simulink model "foc"  (Simulink 5.0)
settings: Solver=ode5  StartTime=0.0  StopTime=3  FixedStep=0.00001  RelTol=1e-3
settings Model: LastModifiedBy=Administrator

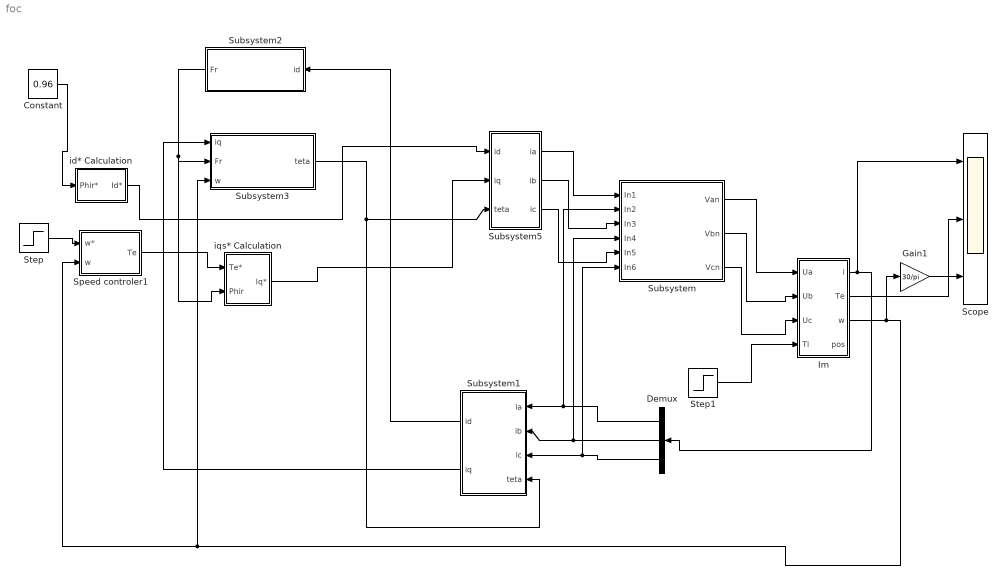
== system foc ==
  Constant : Constant  Value=0.96
  Demux : Demux  Orientation=left  Outputs=3
  Gain1 : Gain  Gain=30/pi  SaturateOnIntegerOverflow=on
  Im : Subsystem  mask{Rs=4.1, Rr=2.5, Ls=0.545, Lr=0.542, Lm=0.510, J=0.04, p=2, Lsc=0.065}
      mask prompts: Rs "stator r(Rs)"; Rr "rotor r(Rr)"; Ls "stator l(Ls)"; Lr "rotor l(Lr)"; Lm "s r l(Lm)"; J "z(J)"; p "jiduishu(p)"; Lsc "l(Lsc)"
  Scope : Scope  NumInputPorts=3
      settings: TimeRange=3  YMin=-12.5~-15~500  YMax=12.5~15~2500  MaxDataPoints=5000000
  Speed controler1 : Subsystem  mask{Kp=30, Ki=5}
  Step : Step  Before=250  After=150  SampleTime=0
  Step1 : Step  Time=2  After=5  SampleTime=0
  Subsystem : Subsystem  mask{Vd=780}
  Subsystem1 : Subsystem  Orientation=left
  Subsystem2 : Subsystem  Orientation=left  mask{Lr=0.542, Lm=0.510, Rr=2.5}
  Subsystem3 : Subsystem  mask{Lr=0.542, Lm=0.510, Rr=2.5}
  Subsystem5 : Subsystem
  id* Calculation : Subsystem
  iqs* Calculation : Subsystem
  wires:
  Demux/1 -> Subsystem1/1(ia), Subsystem/2(In2)
  Demux/2 -> Subsystem1/2(ib), Subsystem/4(In4)
  Demux/3 -> Subsystem1/3(ic), Subsystem/6(In6)
  Subsystem2/1(Fr) -> Subsystem3/2(Fr), iqs* Calculation/2(Phir)
  Subsystem1/2(iq) -> Subsystem3/1(iq)
  Subsystem1/1(id) -> Subsystem2/1(id)
  Subsystem3/1(teta) -> Subsystem1/4(teta), Subsystem5/3(teta)
  iqs* Calculation/1(Iq*) -> Subsystem5/2(iq)
  Subsystem5/1(ia) -> Subsystem/1(In1)
  Subsystem5/2(ib) -> Subsystem/3(In3)
  Subsystem5/3(ic) -> Subsystem/5(In5)
  Subsystem/1(Van) -> Im/1(Ua)
  Subsystem/2(Vbn) -> Im/2(Ub)
  Subsystem/3(Vcn) -> Im/3(Uc)
  Im/3(w) -> Subsystem3/3(w), Speed controler1/2(w), Gain1/1
  Im/1(i) -> Demux/1, Scope/1
  Constant/1 -> id* Calculation/1(Phir*)
  id* Calculation/1(Id*) -> Subsystem5/1(id)
  Step/1 -> Speed controler1/1(w*)
  Im/2(Te) -> Scope/2
  Step1/1 -> Im/4(Tl)
  Speed controler1/1(Te) -> iqs* Calculation/1(Te*)
  Gain1/1 -> Scope/3

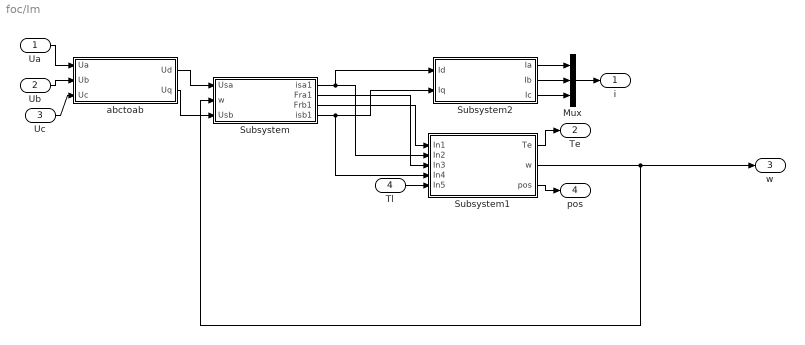
== system foc/Im ==
  Ua : Inport
  Ub : Inport  Port=2
  Uc : Inport  Port=3
  Tl : Inport  Port=4
  Mux : Mux  Inputs=3
  Subsystem : Subsystem
  Subsystem1 : Subsystem
  Subsystem2 : Subsystem
  abctoab : Subsystem
  i : Outport
  Te : Outport  Port=2
  w : Outport  Port=3
  pos : Outport  Port=4
  wires:
  Ua/1 -> abctoab/1(Ua)
  Mux/1 -> i/1
  Ub/1 -> abctoab/2(Ub)
  Uc/1 -> abctoab/3(Uc)
  Subsystem1/1(Te) -> Te/1
  Tl/1 -> Subsystem1/5(In5)
  Subsystem1/3(pos) -> pos/1
  Subsystem1/2(w) -> Subsystem/2(w), w/1
  Subsystem2/3(Ic) -> Mux/3
  Subsystem2/2(Ib) -> Mux/2
  Subsystem2/1(Ia) -> Mux/1
  Subsystem/2(Fra1) -> Subsystem1/3(In3)
  Subsystem/3(Frb1) -> Subsystem1/1(In1)
  Subsystem/4(isb1) -> Subsystem2/2(Iq), Subsystem1/4(In4)
  Subsystem/1(isa1) -> Subsystem2/1(Id), Subsystem1/2(In2)
  abctoab/2(Uq) -> Subsystem/3(Usb)
  abctoab/1(Ud) -> Subsystem/1(Usa)

== system foc/Speed controler1 ==
  w* : Inport
  w : Inport  Port=2
  Gain : Gain  Gain=Kp  SaturateOnIntegerOverflow=on
  Gain1 : Gain  Gain=Ki  SaturateOnIntegerOverflow=on
  Integrator : Integrator
  Saturation : Saturate  UpperLimit=20  LowerLimit=-20
  Sum : Sum  Inputs=|+-  SaturateOnIntegerOverflow=on
  Sum1 : Sum  Inputs=|++  SaturateOnIntegerOverflow=on
  Te : Outport
  wires:
  Sum/1 -> Gain/1, Gain1/1
  Gain1/1 -> Integrator/1
  Integrator/1 -> Sum1/2
  Gain/1 -> Sum1/1
  w*/1 -> Sum/1
  w/1 -> Sum/2
  Sum1/1 -> Saturation/1
  Saturation/1 -> Te/1

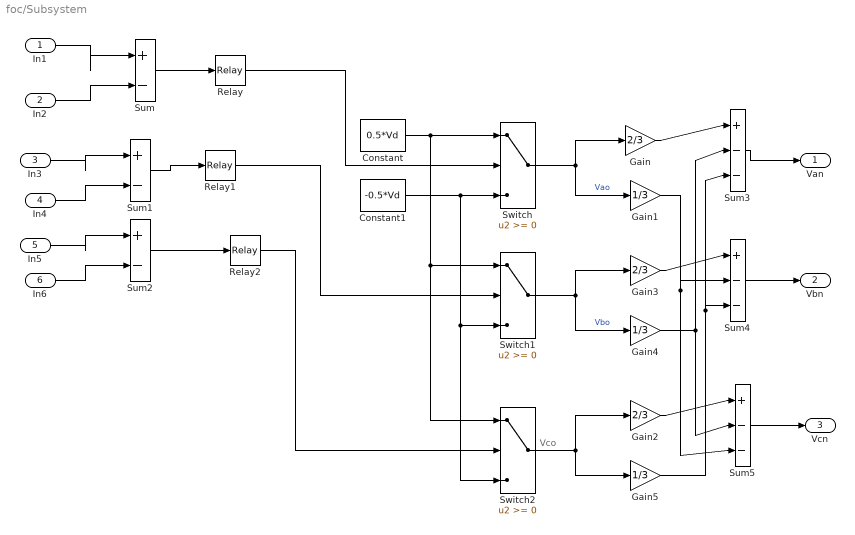
== system foc/Subsystem ==
  note: Vco
  In1 : Inport
  In2 : Inport  Port=2
  In3 : Inport  Port=3
  In4 : Inport  Port=4
  In5 : Inport  Port=5
  In6 : Inport  Port=6
  Constant : Constant  Value=0.5*Vd
  Constant1 : Constant  Value=-0.5*Vd
  Gain : Gain  Gain=2/3  SaturateOnIntegerOverflow=on
  Gain1 : Gain  Gain=1/3  SaturateOnIntegerOverflow=on
  Gain2 : Gain  Gain=2/3  SaturateOnIntegerOverflow=on
  Gain3 : Gain  Gain=2/3  SaturateOnIntegerOverflow=on
  Gain4 : Gain  Gain=1/3  SaturateOnIntegerOverflow=on
  Gain5 : Gain  Gain=1/3  SaturateOnIntegerOverflow=on
  Relay : Relay  OnSwitchValue=0.001  OffSwitchValue=-0.001  OffOutputValue=-1
  Relay1 : Relay  OnSwitchValue=0.001  OffSwitchValue=0.001  OffOutputValue=-1
  Relay2 : Relay  OnSwitchValue=0.001  OffSwitchValue=0.001  OffOutputValue=-1
  Sum : Sum  Inputs=|+-  SaturateOnIntegerOverflow=on
  Sum1 : Sum  Inputs=|+-  SaturateOnIntegerOverflow=on
  Sum2 : Sum  Inputs=|+-  SaturateOnIntegerOverflow=on
  Sum3 : Sum  Inputs=|+--  SaturateOnIntegerOverflow=on
  Sum4 : Sum  Inputs=|+--  SaturateOnIntegerOverflow=on
  Sum5 : Sum  Inputs=|+--  SaturateOnIntegerOverflow=on
  Switch : Switch  SaturateOnIntegerOverflow=on
  Switch1 : Switch  SaturateOnIntegerOverflow=on
  Switch2 : Switch  SaturateOnIntegerOverflow=on
  Van : Outport
  Vbn : Outport  Port=2
  Vcn : Outport  Port=3
  wires:
  Sum/1 -> Relay/1
  In1/1 -> Sum/1
  In2/1 -> Sum/2
  In3/1 -> Sum1/1
  In4/1 -> Sum1/2
  In5/1 -> Sum2/1
  In6/1 -> Sum2/2
  Sum2/1 -> Relay2/1
  Sum1/1 -> Relay1/1
  Relay/1 -> Switch/2
  Constant/1 -> Switch/1, Switch2/1, Switch1/1
  Constant1/1 -> Switch/3, Switch2/3, Switch1/3
  Switch/1 -> Gain/1, Gain1/1  "Vao"
  Switch1/1 -> Gain3/1, Gain4/1  "Vbo"
  Switch2/1 -> Gain2/1, Gain5/1
  Sum3/1 -> Van/1
  Sum4/1 -> Vbn/1
  Sum5/1 -> Vcn/1
  Gain/1 -> Sum3/1
  Gain4/1 -> Sum3/2, Sum5/2
  Gain5/1 -> Sum3/3, Sum4/3
  Gain3/1 -> Sum4/1
  Gain1/1 -> Sum4/2, Sum5/3
  Gain2/1 -> Sum5/1
  Relay1/1 -> Switch1/2
  Relay2/1 -> Switch2/2

== system foc/Subsystem1 ==
  ia : Inport
  ib : Inport  Port=2
  ic : Inport  Port=3
  teta : Inport  Port=4
  VR : Subsystem
  abctoab : Subsystem
  id : Outport
  iq : Outport  Port=2
  wires:
  VR/2(Out2) -> iq/1
  VR/1(Out1) -> id/1
  teta/1 -> VR/3(In3)
  ic/1 -> abctoab/3(Uc)
  ib/1 -> abctoab/2(Ub)
  ia/1 -> abctoab/1(Ua)
  abctoab/2(Uq) -> VR/2(In2)
  abctoab/1(Ud) -> VR/1(In1)

== system foc/Subsystem2 ==
  id : Inport
  Gain : Gain  Gain=Lm*Rr  SaturateOnIntegerOverflow=on
  Transfer Fcn : TransferFcn  Denominator=[Lr Rr]
  Fr : Outport
  wires:
  Transfer Fcn/1 -> Fr/1
  Gain/1 -> Transfer Fcn/1
  id/1 -> Gain/1

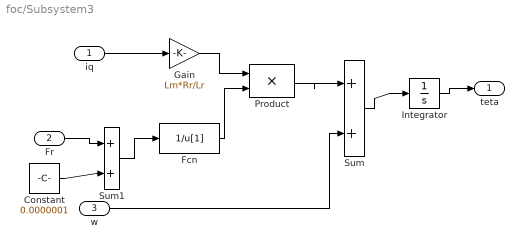
== system foc/Subsystem3 ==
  iq : Inport
  Fr : Inport  Port=2
  w : Inport  Port=3
  Constant : Constant  Value=0.0000001
  Fcn : Fcn  Expr=1/u[1]
  Gain : Gain  Gain=Lm*Rr/Lr  SaturateOnIntegerOverflow=on
  Integrator : Integrator
  Product : Product  SaturateOnIntegerOverflow=on
  Sum : Sum  Inputs=|++  SaturateOnIntegerOverflow=on
  Sum1 : Sum  Inputs=|++  SaturateOnIntegerOverflow=on
  teta : Outport
  wires:
  Product/1 -> Sum/1
  Fcn/1 -> Product/2
  Gain/1 -> Product/1
  iq/1 -> Gain/1
  Sum/1 -> Integrator/1
  Integrator/1 -> teta/1
  w/1 -> Sum/2
  Constant/1 -> Sum1/2
  Fr/1 -> Sum1/1
  Sum1/1 -> Fcn/1

== system foc/Subsystem5 ==
  id : Inport
  iq : Inport  Port=2
  teta : Inport  Port=3
  Subsystem2 : Subsystem
  VR-1 : Subsystem
  ia : Outport
  ib : Outport  Port=2
  ic : Outport  Port=3
  wires:
  Subsystem2/3(Ic) -> ic/1
  Subsystem2/2(Ib) -> ib/1
  Subsystem2/1(Ia) -> ia/1
  teta/1 -> VR-1/3(teta)
  iq/1 -> VR-1/2(iq)
  id/1 -> VR-1/1(id)
  VR-1/2(ib) -> Subsystem2/2(Iq)
  VR-1/1(ia) -> Subsystem2/1(Id)

== system foc/id* Calculation ==
  note: Id* = Phir*/ Lm
  note: Lm= 34.7 mH
  Phir* : Inport
  KF : Gain  Gain=1/0.51  SaturateOnIntegerOverflow=on
  Id* : Outport
  wires:
  KF/1 -> Id*/1
  Phir*/1 -> KF/1

== system foc/iqs* Calculation ==
  note: Iq= ( 2/3) * (2/p) * ( Lr/Lm) * (Te / Phir)
  note: Lm = 34.7 mH
  note: Lr = Ll'r +Lm = 0.8 +34.7= 35.5 mH
  note: p= nb of poles = 4
  note: Iq= 0.341 * (Te / Phir)
  Te* : Inport
  Phir : Inport  Port=2
  Fcn : Fcn  Expr=u[1]*0.341/(u[2]+1e-3)
  Mux1 : Mux  Inputs=2
  Iq* : Outport  InitialOutput=0
  wires:
  Phir/1 -> Mux1/2
  Fcn/1 -> Iq*/1
  Te*/1 -> Mux1/1
  Mux1/1 -> Fcn/1

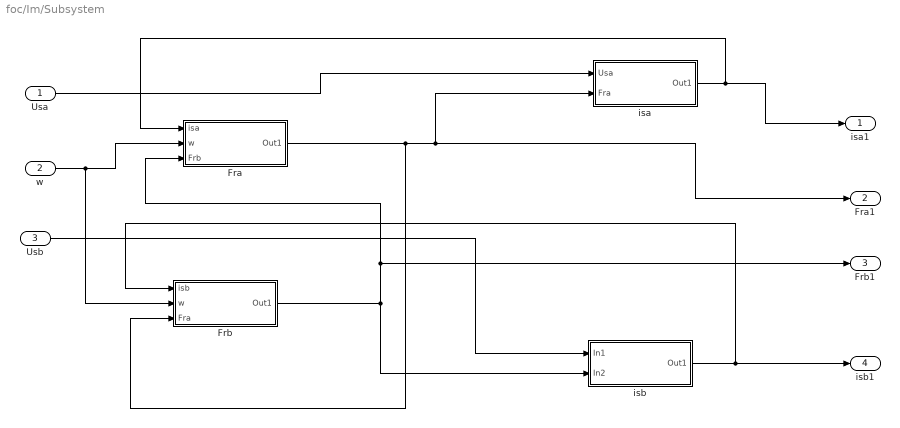
== system foc/Im/Subsystem ==
  Usa : Inport
  w : Inport  Port=2
  Usb : Inport  Port=3
  Fra : Subsystem
  Frb : Subsystem
  isa : Subsystem
  isb : Subsystem
  isa1 : Outport
  Fra1 : Outport  Port=2
  Frb1 : Outport  Port=3
  isb1 : Outport  Port=4
  wires:
  Usa/1 -> isa/1(Usa)
  Fra/1(Out1) -> Frb/3(Fra), isa/2(Fra), Fra1/1
  isa/1(Out1) -> isa1/1, Fra/1(isa)
  w/1 -> Fra/2(w), Frb/2(w)
  Frb/1(Out1) -> isb/2(In2), Fra/3(Frb), Frb1/1
  Usb/1 -> isb/1(In1)
  isb/1(Out1) -> Frb/1(isb), isb1/1

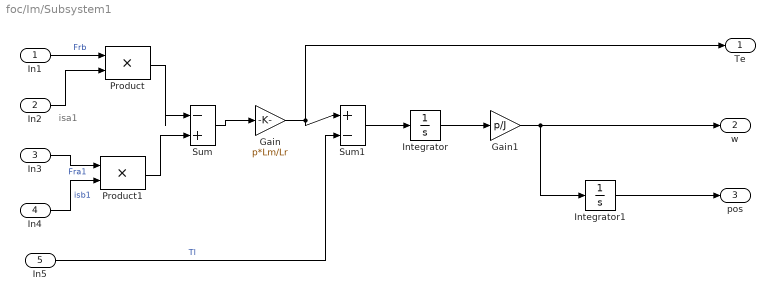
== system foc/Im/Subsystem1 ==
  note: isa1
  In1 : Inport
  In2 : Inport  Port=2
  In3 : Inport  Port=3
  In4 : Inport  Port=4
  In5 : Inport  Port=5
  Gain : Gain  Gain=p*Lm/Lr  SaturateOnIntegerOverflow=on
  Gain1 : Gain  Gain=p/J  SaturateOnIntegerOverflow=on
  Integrator : Integrator
  Integrator1 : Integrator
  Product : Product  SaturateOnIntegerOverflow=on
  Product1 : Product  SaturateOnIntegerOverflow=on
  Sum : Sum  Inputs=|-+  SaturateOnIntegerOverflow=on
  Sum1 : Sum  Inputs=|+-  SaturateOnIntegerOverflow=on
  Te : Outport
  w : Outport  Port=2
  pos : Outport  Port=3
  wires:
  In1/1 -> Product/1  "Frb"
  In2/1 -> Product/2
  In3/1 -> Product1/1  "Fra1"
  In4/1 -> Product1/2  "isb1"
  Product/1 -> Sum/1
  Product1/1 -> Sum/2
  Sum/1 -> Gain/1
  Gain/1 -> Sum1/1, Te/1
  In5/1 -> Sum1/2  "Tl"
  Sum1/1 -> Integrator/1
  Integrator/1 -> Gain1/1
  Gain1/1 -> w/1, Integrator1/1
  Integrator1/1 -> pos/1

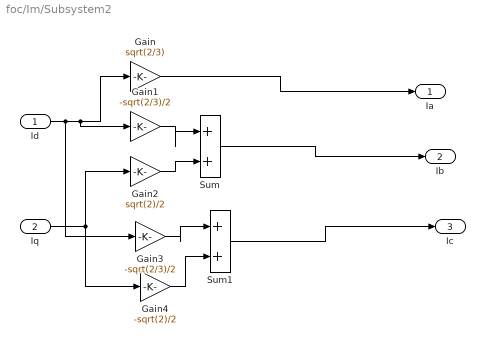
== system foc/Im/Subsystem2 ==
  Id : Inport
  Iq : Inport  Port=2
  Gain : Gain  Gain=sqrt(2/3)  SaturateOnIntegerOverflow=on
  Gain1 : Gain  Gain=-sqrt(2/3)/2  SaturateOnIntegerOverflow=on
  Gain2 : Gain  Gain=sqrt(2)/2  SaturateOnIntegerOverflow=on
  Gain3 : Gain  Gain=-sqrt(2/3)/2  SaturateOnIntegerOverflow=on
  Gain4 : Gain  Gain=-sqrt(2)/2  SaturateOnIntegerOverflow=on
  Sum : Sum  Inputs=|++  SaturateOnIntegerOverflow=on
  Sum1 : Sum  Inputs=|++  SaturateOnIntegerOverflow=on
  Ia : Outport
  Ib : Outport  Port=2
  Ic : Outport  Port=3
  wires:
  Sum1/1 -> Ic/1
  Gain4/1 -> Sum1/2
  Gain3/1 -> Sum1/1
  Sum/1 -> Ib/1
  Gain2/1 -> Sum/2
  Gain1/1 -> Sum/1
  Iq/1 -> Gain4/1, Gain2/1
  Gain/1 -> Ia/1
  Id/1 -> Gain3/1, Gain1/1, Gain/1

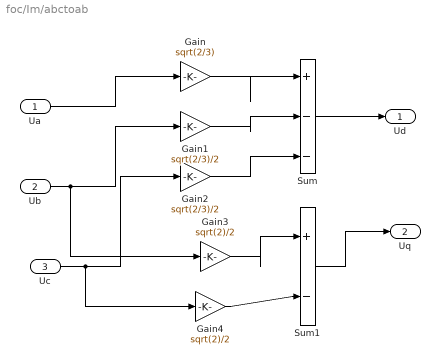
== system foc/Im/abctoab ==
  Ua : Inport
  Ub : Inport  Port=2
  Uc : Inport  Port=3
  Gain : Gain  Gain=sqrt(2/3)  SaturateOnIntegerOverflow=on
  Gain1 : Gain  Gain=sqrt(2/3)/2  SaturateOnIntegerOverflow=on
  Gain2 : Gain  Gain=sqrt(2/3)/2  SaturateOnIntegerOverflow=on
  Gain3 : Gain  Gain=sqrt(2)/2  SaturateOnIntegerOverflow=on
  Gain4 : Gain  Gain=sqrt(2)/2  SaturateOnIntegerOverflow=on
  Sum : Sum  Inputs=|+--  SaturateOnIntegerOverflow=on
  Sum1 : Sum  Inputs=|+-  SaturateOnIntegerOverflow=on
  Ud : Outport
  Uq : Outport  Port=2
  wires:
  Sum1/1 -> Uq/1
  Gain4/1 -> Sum1/2
  Gain3/1 -> Sum1/1
  Sum/1 -> Ud/1
  Gain2/1 -> Sum/3
  Gain1/1 -> Sum/2
  Gain/1 -> Sum/1
  Uc/1 -> Gain4/1, Gain2/1
  Ub/1 -> Gain3/1, Gain1/1
  Ua/1 -> Gain/1

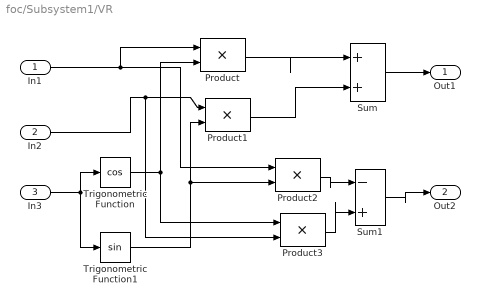
== system foc/Subsystem1/VR ==
  In1 : Inport
  In2 : Inport  Port=2
  In3 : Inport  Port=3
  Product{,1..3} (4 alike) : Product  SaturateOnIntegerOverflow=on
  Sum : Sum  Inputs=|++  SaturateOnIntegerOverflow=on
  Sum1 : Sum  Inputs=|-+  SaturateOnIntegerOverflow=on
  Trigonometric Function : Trigonometry  Operator=cos
  Trigonometric Function1 : Trigonometry
  Out1 : Outport
  Out2 : Outport  Port=2
  wires:
  Product3/1 -> Sum1/2
  Product2/1 -> Sum1/1
  Product1/1 -> Sum/2
  In2/1 -> Product3/2, Product1/1
  Trigonometric Function1/1 -> Product2/2, Product1/2
  Product/1 -> Sum/1
  Trigonometric Function/1 -> Product3/1, Product/2
  In1/1 -> Product2/1, Product/1
  Sum1/1 -> Out2/1
  In3/1 -> Trigonometric Function1/1, Trigonometric Function/1
  Sum/1 -> Out1/1

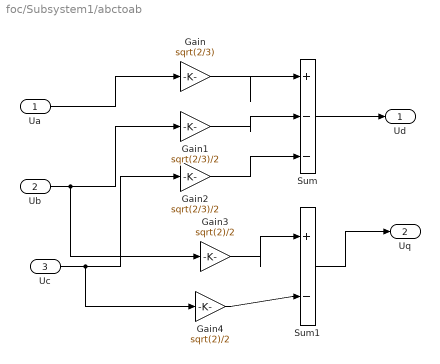
== system foc/Subsystem1/abctoab ==
  Ua : Inport
  Ub : Inport  Port=2
  Uc : Inport  Port=3
  Gain : Gain  Gain=sqrt(2/3)  SaturateOnIntegerOverflow=on
  Gain1 : Gain  Gain=sqrt(2/3)/2  SaturateOnIntegerOverflow=on
  Gain2 : Gain  Gain=sqrt(2/3)/2  SaturateOnIntegerOverflow=on
  Gain3 : Gain  Gain=sqrt(2)/2  SaturateOnIntegerOverflow=on
  Gain4 : Gain  Gain=sqrt(2)/2  SaturateOnIntegerOverflow=on
  Sum : Sum  Inputs=|+--  SaturateOnIntegerOverflow=on
  Sum1 : Sum  Inputs=|+-  SaturateOnIntegerOverflow=on
  Ud : Outport
  Uq : Outport  Port=2
  wires:
  Sum1/1 -> Uq/1
  Gain4/1 -> Sum1/2
  Gain3/1 -> Sum1/1
  Sum/1 -> Ud/1
  Gain2/1 -> Sum/3
  Gain1/1 -> Sum/2
  Gain/1 -> Sum/1
  Uc/1 -> Gain4/1, Gain2/1
  Ub/1 -> Gain3/1, Gain1/1
  Ua/1 -> Gain/1

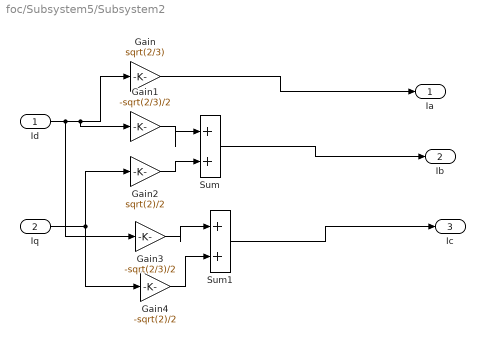
== system foc/Subsystem5/Subsystem2 ==
  Id : Inport
  Iq : Inport  Port=2
  Gain : Gain  Gain=sqrt(2/3)  SaturateOnIntegerOverflow=on
  Gain1 : Gain  Gain=-sqrt(2/3)/2  SaturateOnIntegerOverflow=on
  Gain2 : Gain  Gain=sqrt(2)/2  SaturateOnIntegerOverflow=on
  Gain3 : Gain  Gain=-sqrt(2/3)/2  SaturateOnIntegerOverflow=on
  Gain4 : Gain  Gain=-sqrt(2)/2  SaturateOnIntegerOverflow=on
  Sum : Sum  Inputs=|++  SaturateOnIntegerOverflow=on
  Sum1 : Sum  Inputs=|++  SaturateOnIntegerOverflow=on
  Ia : Outport
  Ib : Outport  Port=2
  Ic : Outport  Port=3
  wires:
  Id/1 -> Gain/1, Gain1/1, Gain3/1
  Gain/1 -> Ia/1
  Iq/1 -> Gain2/1, Gain4/1
  Gain1/1 -> Sum/1
  Gain2/1 -> Sum/2
  Sum/1 -> Ib/1
  Gain3/1 -> Sum1/1
  Gain4/1 -> Sum1/2
  Sum1/1 -> Ic/1

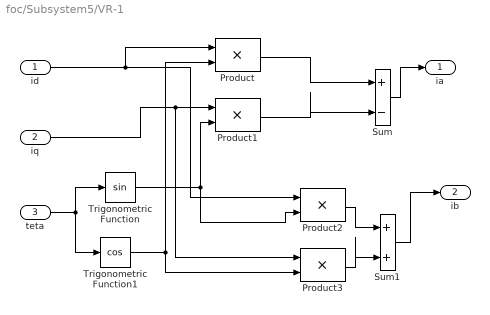
== system foc/Subsystem5/VR-1 ==
  id : Inport
  iq : Inport  Port=2
  teta : Inport  Port=3
  Product{,1..3} (4 alike) : Product  SaturateOnIntegerOverflow=on
  Sum : Sum  Inputs=|+-  SaturateOnIntegerOverflow=on
  Sum1 : Sum  Inputs=|++  SaturateOnIntegerOverflow=on
  Trigonometric Function : Trigonometry
  Trigonometric Function1 : Trigonometry  Operator=cos
  ia : Outport
  ib : Outport  Port=2
  wires:
  Sum1/1 -> ib/1
  Product3/1 -> Sum1/2
  Product2/1 -> Sum1/1
  Sum/1 -> ia/1
  Product1/1 -> Sum/2
  iq/1 -> Product3/1, Product1/1
  Trigonometric Function/1 -> Product2/2, Product1/2
  Product/1 -> Sum/1
  Trigonometric Function1/1 -> Product3/2, Product/2
  id/1 -> Product2/1, Product/1
  teta/1 -> Trigonometric Function1/1, Trigonometric Function/1

== system foc/Im/Subsystem/Fra ==
  isa : Inport
  w : Inport  Port=2
  Frb : Inport  Port=3
  Gain : Gain  Gain=Lm*Rr  SaturateOnIntegerOverflow=on
  Gain1 : Gain  Gain=Lr  SaturateOnIntegerOverflow=on
  Product : Product  SaturateOnIntegerOverflow=on
  Sum : Sum  Inputs=|+-  SaturateOnIntegerOverflow=on
  Transfer Fcn : TransferFcn  Denominator=[Lr Rr]
  Out1 : Outport
  wires:
  isa/1 -> Gain/1
  Frb/1 -> Gain1/1
  Gain1/1 -> Product/2
  w/1 -> Product/1
  Gain/1 -> Sum/1
  Product/1 -> Sum/2
  Sum/1 -> Transfer Fcn/1
  Transfer Fcn/1 -> Out1/1

== system foc/Im/Subsystem/Frb ==
  isb : Inport
  w : Inport  Port=2
  Fra : Inport  Port=3
  Gain : Gain  Gain=Lm*Rr  SaturateOnIntegerOverflow=on
  Gain1 : Gain  Gain=Lr  SaturateOnIntegerOverflow=on
  Product : Product  SaturateOnIntegerOverflow=on
  Sum : Sum  Inputs=|++  SaturateOnIntegerOverflow=on
  Transfer Fcn : TransferFcn  Denominator=[Lr Rr]
  Out1 : Outport
  wires:
  isb/1 -> Gain/1
  Gain/1 -> Sum/1
  Fra/1 -> Gain1/1
  Gain1/1 -> Product/2
  w/1 -> Product/1
  Product/1 -> Sum/2
  Sum/1 -> Transfer Fcn/1
  Transfer Fcn/1 -> Out1/1

== system foc/Im/Subsystem/isa ==
  Usa : Inport
  Fra : Inport  Port=2
  Gain : Gain  Gain=1/Lr  SaturateOnIntegerOverflow=on
  Sum : Sum  Inputs=|+-  SaturateOnIntegerOverflow=on
  Transfer Fcn : TransferFcn  Denominator=[Lsc Rs]
  Transfer Fcn1 : TransferFcn  Numerator=[Lm 0]  Denominator=[Lsc Rs]
  Out1 : Outport
  wires:
  Usa/1 -> Transfer Fcn/1
  Fra/1 -> Gain/1
  Gain/1 -> Transfer Fcn1/1
  Transfer Fcn1/1 -> Sum/2
  Transfer Fcn/1 -> Sum/1
  Sum/1 -> Out1/1

== system foc/Im/Subsystem/isb ==
  In1 : Inport
  In2 : Inport  Port=2
  Gain : Gain  Gain=1/Lr  SaturateOnIntegerOverflow=on
  Sum : Sum  Inputs=|+-  SaturateOnIntegerOverflow=on
  Transfer Fcn : TransferFcn  Denominator=[Lsc Rs]
  Transfer Fcn1 : TransferFcn  Numerator=[Lm 0]  Denominator=[Lsc Rs]
  Out1 : Outport
  wires:
  In2/1 -> Gain/1
  Gain/1 -> Transfer Fcn1/1
  Transfer Fcn1/1 -> Sum/2
  In1/1 -> Transfer Fcn/1
  Transfer Fcn/1 -> Sum/1
  Sum/1 -> Out1/1
